simulink model "model_ref_liblink"  (Simulink 7.9)
settings: Solver=FixedStepDiscrete  StartTime=0.0  StopTime=10.0  FixedStep=1  RelTol=1e-3
PreLoadFcn:
  | if exist('tl_preloadfcn','file'), tl_preloadfcn(gcs,101); end
PostLoadFcn:
  | if exist('tl_postloadfcn','file'), tl_postloadfcn(gcs,101); end
InitFcn:
  | if exist('tlds_init','file'), tlds_init(gcs); end
StartFcn:
  | if exist('tlds_start','file'), tlds_start(gcs); end
StopFcn:
  | if exist('tlds_stop','file'), tlds_stop(gcs); end
libraries: tllib x5, model_ref_lib x1
PreSaveFcn:
  | if exist('tl_presavefcn','file'), tl_presavefcn(gcs); end
settings Model: TL_MAIN_DATA={'#advcodeopt',0,'logopt',{'mdlrefmode',2},'date',736211.63933920139}  TLRevision=101  DS_PROJECTFILE=model_ref.dd  DS_APPLICATION=model_ref  Creator=Administrator  LastModifiedBy=developer  BufferReuse=off
settings OptimizationCC: BlockReduction=off  OptimizeBlockIOStorage=off  BufferReuse=off  ExpressionFolding=off  LocalBlockOutputs=off  InitFltsAndDblsToZero=on
settings DebuggingCC: SaveWithParameterizedLinksMsg=none  SignalResolutionControl=TryResolveAllWithWarning  MultiTaskDSMMsg=warning  MultiTaskCondExecSysMsg=none  FcnCallInpInsideContextMsg=Use local settings
settings RTWCC: IncludeERTFirstTime=on
settings GRTTargetCC: TargetFcnLib=ansi_tfl_tmw.mat  CombineOutputUpdateFcns=off  GRTInterface=on

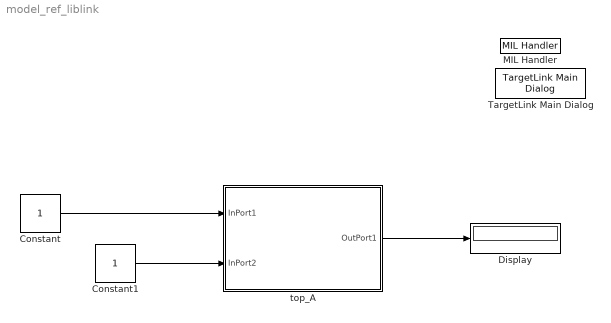
== system model_ref_liblink ==
  Constant : Constant
  Constant1 : Constant
  Display : Display
  MIL Handler : tllib/MIL Handler  data={'date',734678.43845987273}
  TargetLink Main Dialog : tllib/TargetLink Main Dialog  data=[]
  top_A : Subsystem  Tag=TargetLink Simulation Frame
      settings: CopyFcn=if exist('tl_copyfcn','file'), tl_copyfcn(gcbh); end  NameChangeFcn=if exist('tl_framenamechangefcn','file'), tl_framenamechangefcn(gcbh); end
      settings: OpenFcn=|
      | if exist('open_tlsubsystem','file')
      |    open_tlsubsystem(gcbh);
      | else
      |    tlsubsystem = ...
      |       find_system(gcb, ...
      |       'LookUnderMasks','on', ...
      |       'FollowLinks','on', ...
      |       'Tag','MIL Subsystem');
      |    open_system(tlsubsystem);
      | end
      mask Type: TL_SimFrame
      mask Display: disp('TargetLink\nModel-\nin-the-loop\nmode')
  wires:
  Constant/1 -> top_A/1(InPort1)
  top_A/1(OutPort1) -> Display/1
  Constant1/1 -> top_A/2(InPort2)

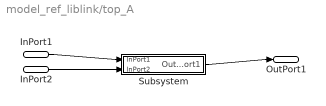
== system model_ref_liblink/top_A ==
  InPort1 : Inport
  InPort2 : Inport  Port=2
  Subsystem : Subsystem  Tag=struct('sfcnName','top_A_sf','subFunction','','srcSubsystem','')
      settings: OpenFcn=warndlg(get_param(gcb,'MaskHelp'),'Serious Warning');
      mask Type: TL_Enable
      mask Help: This subsystem keeps the TargetLink subsystem (subsystem with TargetLink blocks for production code generation), and is needed for the TargetLink simulation frame to work properly. DO NOT DELETE OR MODIFY IT!
  OutPort1 : Outport
  wires:
  InPort1/1 -> Subsystem/1(InPort1)
  InPort2/1 -> Subsystem/2(InPort2)
  Subsystem/1(OutPort1) -> OutPort1/1

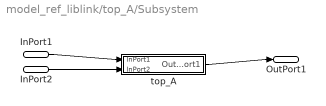
== system model_ref_liblink/top_A/Subsystem ==
  InPort1 : Inport
  InPort2 : Inport  Port=2
  top_A : Subsystem  Tag=MIL Subsystem  Description=a
      settings: CopyFcn=if exist('tl_copyfcn','file'), tl_copyfcn(gcbh); end  NameChangeFcn=if exist('tl_namechangefcn','file'), tl_namechangefcn(gcbh); end  DestroyFcn=if exist('update_tl_main_dlg','file'), update_tl_main_dlg('TL_subs_display'); end
      mask Type: MIL Subsystem
      mask Display: disp('TargetLink Subsystem')
  OutPort1 : Outport
  wires:
  InPort1/1 -> top_A/1(InPort1)
  InPort2/1 -> top_A/2(InPort2)
  top_A/1(OutPort1) -> OutPort1/1

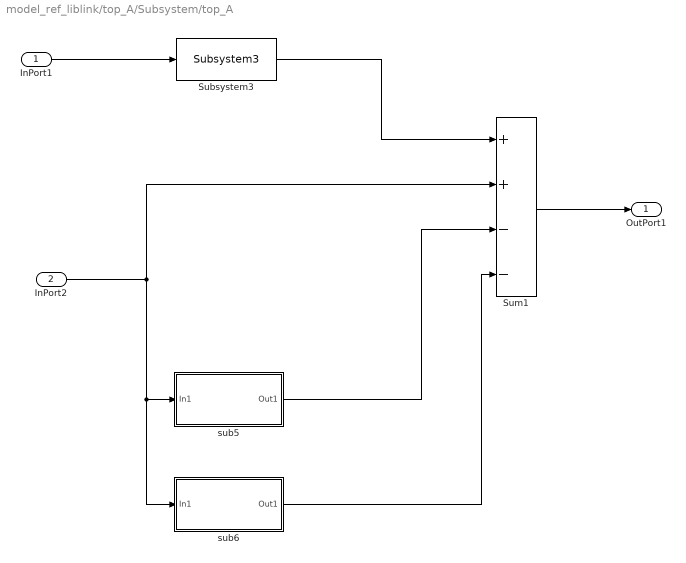
== system model_ref_liblink/top_A/Subsystem/top_A ==
  InPort1 : Inport  mask(TL_Inport){data={'date',734678.43845968752}}
      settings: DeleteFcn=if exist('delete_tlblock','file')==2,delete_tlblock(gcbh);end  OpenFcn=if exist('tl_open_blockdlg','file')==2,tl_open_blockdlg(gcbh);else,open_system(gcbh,'parameter');end
      settings: CopyFcn=|
      | if exist('tl_reset_reviewflag','file')==2
      |     tl_reset_reviewflag(gcbh);
      | end
      | if exist('tl_check_ports','file')
      |     tl_check_ports(gcbh);
      | end
      settings: NameChangeFcn=|
      | if exist('rename_tlblock','file')==2,rename_tlblock(gcbh);end
      | if exist('tl_check_ports','file'), tl_check_ports(gcbh); end
      mask Help: eval(['if exist(''tl_online_help'',''file'') == 2, tl_online_help(''Topic'',''TL_Inport''),else, web([''jar:file:///'',matlabroot,''/help/toolbox/simulink/help.jar!/slref/' lower(get_param(gcbh,'Blocktype')) '.html''], ''-helpbrowser''),end'])
      mask Display: plot([0.2 0.35 NaN 0.65 0.8],[0 1 NaN 0 1]);
  InPort2 : Inport  Port=2  mask(TL_Inport){data={'date',734678.43845932873}}
      settings: DeleteFcn=if exist('delete_tlblock','file')==2,delete_tlblock(gcbh);end  OpenFcn=if exist('tl_open_blockdlg','file')==2,tl_open_blockdlg(gcbh);else,open_system(gcbh,'parameter');end
      settings: CopyFcn=|
      | if exist('tl_reset_reviewflag','file')==2
      |     tl_reset_reviewflag(gcbh);
      | end
      | if exist('tl_check_ports','file')
      |     tl_check_ports(gcbh);
      | end
      settings: NameChangeFcn=|
      | if exist('rename_tlblock','file')==2,rename_tlblock(gcbh);end
      | if exist('tl_check_ports','file'), tl_check_ports(gcbh); end
      mask Help: eval(['if exist(''tl_online_help'',''file'') == 2, tl_online_help(''Topic'',''TL_Inport''),else, web([''jar:file:///'',matlabroot,''/help/toolbox/simulink/help.jar!/slref/' lower(get_param(gcbh,'Blocktype')) '.html''], ''-helpbrowser''),end'])
      mask Display: plot([0.2 0.35 NaN 0.65 0.8],[0 1 NaN 0 1]);
  Subsystem3 : model_ref_lib/Subsystem3
  Sum1 : Sum  Inputs=++--  mask(TL_Sum){data={'date',736211.63795276615}}
      settings: CopyFcn=if exist('tl_reset_reviewflag') == 2, tl_reset_reviewflag(gcbh); end  DeleteFcn=if exist('delete_tlblock','file')==2,delete_tlblock(gcbh);end  NameChangeFcn=if exist('rename_tlblock','file')==2,rename_tlblock(gcbh);end  OpenFcn=if exist('tl_open_blockdlg','file')==2,tl_open_blockdlg(gcbh);else,open_system(gcbh,'parameter');end
      mask Help: eval(['if exist(''tl_online_help'',''file'') == 2, tl_online_help(''Topic'',''TL_Sum''),else, web([''jar:file:///'',matlabroot,''/help/toolbox/simulink/help.jar!/slref/' lower(get_param(gcbh,'Blocktype')) '.html''], ''-helpbrowser''),end'])
      mask Display: plot([-0.05, 1.05, NaN, -0.05, 1.05],[.01, .01, NaN, .99, .99])
  sub5 : Subsystem  TreatAsAtomicUnit=on
  sub6 : Subsystem  TreatAsAtomicUnit=on
  OutPort1 : Outport  mask(TL_Outport){data={'date',734678.43845263892}}
      settings: DeleteFcn=if exist('delete_tlblock','file')==2,delete_tlblock(gcbh);end  OpenFcn=if exist('tl_open_blockdlg','file')==2,tl_open_blockdlg(gcbh);else,open_system(gcbh,'parameter');end
      settings: CopyFcn=|
      | if exist('tl_reset_reviewflag','file')==2
      |     tl_reset_reviewflag(gcbh);
      | end
      | if exist('tl_check_ports','file')
      |     tl_check_ports(gcbh);
      | end
      settings: NameChangeFcn=|
      | if exist('rename_tlblock','file')==2,rename_tlblock(gcbh);end
      | if exist('tl_check_ports','file'), tl_check_ports(gcbh); end
      mask Help: eval(['if exist(''tl_online_help'',''file'') == 2, tl_online_help(''Topic'',''TL_Outport''),else, web([''jar:file:///'',matlabroot,''/help/toolbox/simulink/help.jar!/slref/' lower(get_param(gcbh,'Blocktype')) '.html''], ''-helpbrowser''),end'])
      mask Display: plot([0.2 0.35 NaN 0.65 0.8],[0 1 NaN 0 1]);
  wires:
  Sum1/1 -> OutPort1/1
  InPort2/1 -> sub5/1(In1), sub6/1(In1), Sum1/2
  InPort1/1 -> Subsystem3/1
  Subsystem3/1 -> Sum1/1
  sub5/1(Out1) -> Sum1/3
  sub6/1(Out1) -> Sum1/4

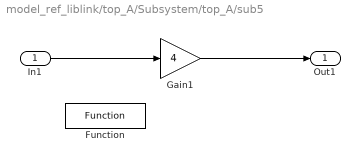
== system model_ref_liblink/top_A/Subsystem/top_A/sub5 ==
  In1 : Inport  mask(TL_Inport){data={'date',734678.43845716433}}
      settings: CopyFcn=if exist('tl_reset_reviewflag','file')==2,tl_reset_reviewflag(gcbh);end  DeleteFcn=if exist('delete_tlblock','file')==2,delete_tlblock(gcbh);end  NameChangeFcn=if exist('rename_tlblock','file')==2,rename_tlblock(gcbh);end  OpenFcn=if exist('tl_open_blockdlg','file')==2,tl_open_blockdlg(gcbh);else,open_system(gcbh,'parameter');end
      mask Help: eval(['if exist(''tl_online_help'',''file'') == 2, tl_online_help(''Topic'',''TL_Inport''),else, web([''jar:file:///'',matlabroot,''/help/toolbox/simulink/help.jar!/slref/' lower(get_param(gcbh,'Blocktype')) '.html''], ''-helpbrowser''),end'])
      mask Display: plot([0.2 0.35 NaN 0.65 0.8],[0 1 NaN 0 1]);
  Function : tllib/Function  data={'stepfunctionname','$S_$I','restartfunctionname','RESTART_$S_$I','initfunctionname','INIT_$S_$I','termfunctionname','TERM_$S_$I','subsystemid','sub5','incrcodegen',1,'date',734678.43845010421}
  Gain1 : Gain  Gain=4  mask(TL_Gain){data={'date',734678.43845679401}}
      settings: CopyFcn=if exist('tl_reset_reviewflag') == 2, tl_reset_reviewflag(gcbh); end  DeleteFcn=if exist('delete_tlblock','file')==2,delete_tlblock(gcbh);end  NameChangeFcn=if exist('rename_tlblock','file')==2,rename_tlblock(gcbh);end  OpenFcn=if exist('tl_open_blockdlg','file')==2,tl_open_blockdlg(gcbh);else,open_system(gcbh,'parameter');end
      mask Help: eval(['if exist(''tl_online_help'',''file'') == 2, tl_online_help(''Topic'',''TL_Gain''),else, web([''jar:file:///'',matlabroot,''/help/toolbox/simulink/help.jar!/slref/' lower(get_param(gcbh,'Blocktype')) '.html''], ''-helpbrowser''),end'])
      mask Display: plot([0, .9, 0],[.05, .5, .95])
  Out1 : Outport  mask(TL_Outport){data={'date',734678.43845643522}}
      settings: CopyFcn=if exist('tl_reset_reviewflag','file')==2,tl_reset_reviewflag(gcbh);end  DeleteFcn=if exist('delete_tlblock','file')==2,delete_tlblock(gcbh);end  NameChangeFcn=if exist('rename_tlblock','file')==2,rename_tlblock(gcbh);end  OpenFcn=if exist('tl_open_blockdlg','file')==2,tl_open_blockdlg(gcbh);else,open_system(gcbh,'parameter');end
      mask Help: eval(['if exist(''tl_online_help'',''file'') == 2, tl_online_help(''Topic'',''TL_Outport''),else, web([''jar:file:///'',matlabroot,''/help/toolbox/simulink/help.jar!/slref/' lower(get_param(gcbh,'Blocktype')) '.html''], ''-helpbrowser''),end'])
      mask Display: plot([0.2 0.35 NaN 0.65 0.8],[0 1 NaN 0 1]);
  wires:
  In1/1 -> Gain1/1
  Gain1/1 -> Out1/1

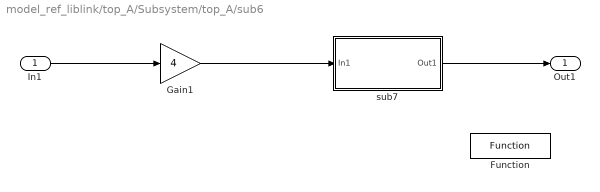
== system model_ref_liblink/top_A/Subsystem/top_A/sub6 ==
  In1 : Inport  mask(TL_Inport){data={'date',734678.43845589121}}
      settings: CopyFcn=if exist('tl_reset_reviewflag','file')==2,tl_reset_reviewflag(gcbh);end  DeleteFcn=if exist('delete_tlblock','file')==2,delete_tlblock(gcbh);end  NameChangeFcn=if exist('rename_tlblock','file')==2,rename_tlblock(gcbh);end  OpenFcn=if exist('tl_open_blockdlg','file')==2,tl_open_blockdlg(gcbh);else,open_system(gcbh,'parameter');end
      mask Help: eval(['if exist(''tl_online_help'',''file'') == 2, tl_online_help(''Topic'',''TL_Inport''),else, web([''jar:file:///'',matlabroot,''/help/toolbox/simulink/help.jar!/slref/' lower(get_param(gcbh,'Blocktype')) '.html''], ''-helpbrowser''),end'])
      mask Display: plot([0.2 0.35 NaN 0.65 0.8],[0 1 NaN 0 1]);
  Function : tllib/Function  data={'subsystemid','sub6','date',734678.43844974542}
  Gain1 : Gain  Gain=4  mask(TL_Gain){data={'date',734678.4384553472}}
      settings: CopyFcn=if exist('tl_reset_reviewflag') == 2, tl_reset_reviewflag(gcbh); end  DeleteFcn=if exist('delete_tlblock','file')==2,delete_tlblock(gcbh);end  NameChangeFcn=if exist('rename_tlblock','file')==2,rename_tlblock(gcbh);end  OpenFcn=if exist('tl_open_blockdlg','file')==2,tl_open_blockdlg(gcbh);else,open_system(gcbh,'parameter');end
      mask Help: eval(['if exist(''tl_online_help'',''file'') == 2, tl_online_help(''Topic'',''TL_Gain''),else, web([''jar:file:///'',matlabroot,''/help/toolbox/simulink/help.jar!/slref/' lower(get_param(gcbh,'Blocktype')) '.html''], ''-helpbrowser''),end'])
      mask Display: plot([0, .9, 0],[.05, .5, .95])
  sub7 : Subsystem  TreatAsAtomicUnit=on
  Out1 : Outport  mask(TL_Outport){data={'date',734678.43845336803}}
      settings: CopyFcn=if exist('tl_reset_reviewflag','file')==2,tl_reset_reviewflag(gcbh);end  DeleteFcn=if exist('delete_tlblock','file')==2,delete_tlblock(gcbh);end  NameChangeFcn=if exist('rename_tlblock','file')==2,rename_tlblock(gcbh);end  OpenFcn=if exist('tl_open_blockdlg','file')==2,tl_open_blockdlg(gcbh);else,open_system(gcbh,'parameter');end
      mask Help: eval(['if exist(''tl_online_help'',''file'') == 2, tl_online_help(''Topic'',''TL_Outport''),else, web([''jar:file:///'',matlabroot,''/help/toolbox/simulink/help.jar!/slref/' lower(get_param(gcbh,'Blocktype')) '.html''], ''-helpbrowser''),end'])
      mask Display: plot([0.2 0.35 NaN 0.65 0.8],[0 1 NaN 0 1]);
  wires:
  Gain1/1 -> sub7/1(In1)
  In1/1 -> Gain1/1
  sub7/1(Out1) -> Out1/1

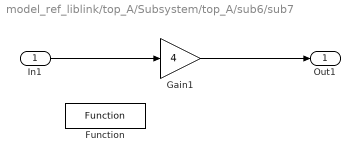
== system model_ref_liblink/top_A/Subsystem/top_A/sub6/sub7 ==
  In1 : Inport  mask(TL_Inport){data={'date',734678.43845498841}}
      settings: CopyFcn=if exist('tl_reset_reviewflag','file')==2,tl_reset_reviewflag(gcbh);end  DeleteFcn=if exist('delete_tlblock','file')==2,delete_tlblock(gcbh);end  NameChangeFcn=if exist('rename_tlblock','file')==2,rename_tlblock(gcbh);end  OpenFcn=if exist('tl_open_blockdlg','file')==2,tl_open_blockdlg(gcbh);else,open_system(gcbh,'parameter');end
      mask Help: eval(['if exist(''tl_online_help'',''file'') == 2, tl_online_help(''Topic'',''TL_Inport''),else, web([''jar:file:///'',matlabroot,''/help/toolbox/simulink/help.jar!/slref/' lower(get_param(gcbh,'Blocktype')) '.html''], ''-helpbrowser''),end'])
      mask Display: plot([0.2 0.35 NaN 0.65 0.8],[0 1 NaN 0 1]);
  Function : tllib/Function  data={'stepfunctionname','$S_$I','restartfunctionname','RESTART_$S_$I','initfunctionname','INIT_$S_$I','termfunctionname','TERM_$S_$I','subsystemid','sub7','incrcodegen',1,'date',734678.43844758102}
  Gain1 : Gain  Gain=4  mask(TL_Gain){data={'date',734678.4384544444}}
      settings: CopyFcn=if exist('tl_reset_reviewflag') == 2, tl_reset_reviewflag(gcbh); end  DeleteFcn=if exist('delete_tlblock','file')==2,delete_tlblock(gcbh);end  NameChangeFcn=if exist('rename_tlblock','file')==2,rename_tlblock(gcbh);end  OpenFcn=if exist('tl_open_blockdlg','file')==2,tl_open_blockdlg(gcbh);else,open_system(gcbh,'parameter');end
      mask Help: eval(['if exist(''tl_online_help'',''file'') == 2, tl_online_help(''Topic'',''TL_Gain''),else, web([''jar:file:///'',matlabroot,''/help/toolbox/simulink/help.jar!/slref/' lower(get_param(gcbh,'Blocktype')) '.html''], ''-helpbrowser''),end'])
      mask Display: plot([0, .9, 0],[.05, .5, .95])
  Out1 : Outport  mask(TL_Outport){data={'date',734678.43845372682}}
      settings: CopyFcn=if exist('tl_reset_reviewflag','file')==2,tl_reset_reviewflag(gcbh);end  DeleteFcn=if exist('delete_tlblock','file')==2,delete_tlblock(gcbh);end  NameChangeFcn=if exist('rename_tlblock','file')==2,rename_tlblock(gcbh);end  OpenFcn=if exist('tl_open_blockdlg','file')==2,tl_open_blockdlg(gcbh);else,open_system(gcbh,'parameter');end
      mask Help: eval(['if exist(''tl_online_help'',''file'') == 2, tl_online_help(''Topic'',''TL_Outport''),else, web([''jar:file:///'',matlabroot,''/help/toolbox/simulink/help.jar!/slref/' lower(get_param(gcbh,'Blocktype')) '.html''], ''-helpbrowser''),end'])
      mask Display: plot([0.2 0.35 NaN 0.65 0.8],[0 1 NaN 0 1]);
  wires:
  Gain1/1 -> Out1/1
  In1/1 -> Gain1/1
